simulink model "slx3_step15_obsv_fb-1"  (R2017b)
settings: Solver=ode45  StartTime=0.0  StopTime=10.0  RelTol=1e-3  EnableMultiTasking=on
values from neighbouring files (symbols this model uses):
  A = sys.A    [fn6_state_estimator-1.m]    (also in fn7_feedback-1.m; fn8_obsv_feedback-1.m; main_function-1.m = [a11 a12 a13 a14)
  B = sys.B    [fn6_state_estimator-1.m]    (also in fn7_feedback-1.m; fn8_obsv_feedback-1.m; main_function-1.m = [0)
  C = sys.C    [fn6_state_estimator-1.m]    (also in fn7_feedback-1.m; fn8_obsv_feedback-1.m; main_function-1.m = eye(size(A)))
  D = sys.D    [fn6_state_estimator-1.m]    (also in fn7_feedback-1.m; fn8_obsv_feedback-1.m; main_function-1.m = zeros(size(B)))
  K = place(A, B, P1)    [fn7_feedback-1.m]
  L = transpose(L)    [fn6_state_estimator-1.m]    (also in main_function-1.m = fn6_state_estimator(sys_ss,P1,xini,xinihat))
  xini = [0;0;0;0]    [main_function-1.m]
  xinihat = xini    [fn8_obsv_feedback-1.m]    (also in main_function-1.m)
settings Model: Creator=mo114c  LastModifiedBy=anusha7
settings DataIOCC: LimitDataPoints=on  SaveFormat=Array
settings OptimizationCC: LifeSpan=inf
settings DebuggingCC: UnderspecifiedInitializationDetection=Classic  MergeDetectMultiDrivingBlocksExec=none  StateNameClashWarn=warning  SFUnexpectedBacktrackingDiag=warning  SFNoUnconditionalDefaultTransitionDiag=warning  SFExecutionAtInitializationDiag=none
settings HardwareCC: ProdBitPerPointer=32  ProdBitPerSizeT=32  ProdBitPerPtrDiffT=32  ProdLargestAtomicFloat=None  ProdIntDivRoundTo=Undefined  ProdEndianess=Unspecified  ProdWordSize=32  ProdHWDeviceType=32-bit Generic
settings ModelReferenceCC: PropagateSignalLabelsOutOfModel=off
settings CodeAppCC: StateflowObjectComments=on
settings GRTTargetCC: TargetLangStandard=C89/C90 (ANSI)  GeneratePreprocessorConditionals=Disable all
settings ConfigComp: CovMetricSettings=dw  CovHtmlReporting=on  CovSaveCumulativeToWorkspaceVar=on  CovSaveSingleToWorkspaceVar=on  CovExternalEMLEnable=off  CovSFcnEnable=off

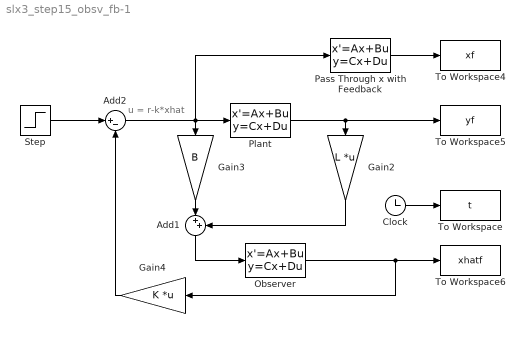
== system slx3_step15_obsv_fb-1 ==
  note: u = r-k*xhat
  Add1 : Sum  Inputs=|++
  Add2 : Sum  Inputs=|+-
  Clock : Clock
  Gain2 : Gain  Gain=L  Multiplication=Matrix(K*u)
  Gain3 : Gain  Gain=B
  Gain4 : Gain  Gain=K  Multiplication=Matrix(K*u)
  Observer : StateSpace  A=A-L*C  B=eye(size(A))  C=eye(size(A))  D=zeros(size(A))  InitialCondition=xinihat
  Pass Through x with Feedback : StateSpace  A=A  B=B  C=eye(size(A))  D=zeros(size(C,1),size(B,2))  InitialCondition=xini
  Plant : StateSpace  A=A  B=B  C=C  D=D  InitialCondition=xini
  Step : Step  Time=0  SampleTime=0
  To Workspace : ToWorkspace  VariableName=t  SampleTime=-1
  To Workspace4 : ToWorkspace  VariableName=xf  SampleTime=-1
  To Workspace5 : ToWorkspace  VariableName=yf  SampleTime=-1
  To Workspace6 : ToWorkspace  VariableName=xhatf  SampleTime=-1
  wires:
  Clock/1 -> To Workspace/1
  Step/1 -> Add2/1
  Add2/1 -> Pass Through x with Feedback/1, Plant/1, Gain3/1
  Pass Through x with Feedback/1 -> To Workspace4/1
  Plant/1 -> To Workspace5/1, Gain2/1
  Gain2/1 -> Add1/2
  Gain3/1 -> Add1/1
  Add1/1 -> Observer/1
  Observer/1 -> To Workspace6/1, Gain4/1
  Gain4/1 -> Add2/2
